simulink library "ECO_TestLibs"  (R2018a)
settings: Solver=ode45  StartTime=0.0  StopTime=10.0  RelTol=1e-3  EnableMultiTasking=on
undefined symbols (not defined in the file or in its folder): h, km
libraries: CoderSF_BSW_Libs x643, $bdroot x217, SF_CanService_Libs x60, simulink x12
(part 5 of 7)

== system ECO_TestLibs/TAF_TRI/FC_L50ms ==
  function : TriggerPort  TriggerType=function-call  VariantControl=(inherit)
  Display : Display
  GetPeriod_ms : $bdroot/GetPeriod_ms  frqP=TRI_frqFreeSys_val
  Write Measurement : CoderSF_BSW_Libs/Calibration & Measurement/Write Measurement  variable_name=TRI_tL50ms  variable_value=0  variable_type=single  numD=1  unitStr=ms  descStr=""
      settings: AttributesFormatString=value:%<variable_value> type:%<variable_type>  SourceProductName=EcoCoder Blocks
  dt : CoderSF_BSW_Libs/Application Base Blocks/dt
      settings: SourceProductName=EcoCoder Blocks
  wires:
  GetPeriod_ms/1 -> Write Measurement/1
  dt/1 -> Display/1

== system ECO_TestLibs/TAF_TRI/FC_L5ms ==
  function : TriggerPort  TriggerType=function-call  VariantControl=(inherit)
  Display : Display
  GetPeriod_ms : $bdroot/GetPeriod_ms  frqP=TRI_frqFreeSys_val
  Write Measurement : CoderSF_BSW_Libs/Calibration & Measurement/Write Measurement  variable_name=TRI_tL5ms  variable_value=0  variable_type=single  numD=1  unitStr=ms  descStr=""
      settings: AttributesFormatString=value:%<variable_value> type:%<variable_type>  SourceProductName=EcoCoder Blocks
  dt : CoderSF_BSW_Libs/Application Base Blocks/dt
      settings: SourceProductName=EcoCoder Blocks
  wires:
  GetPeriod_ms/1 -> Write Measurement/1
  dt/1 -> Display/1

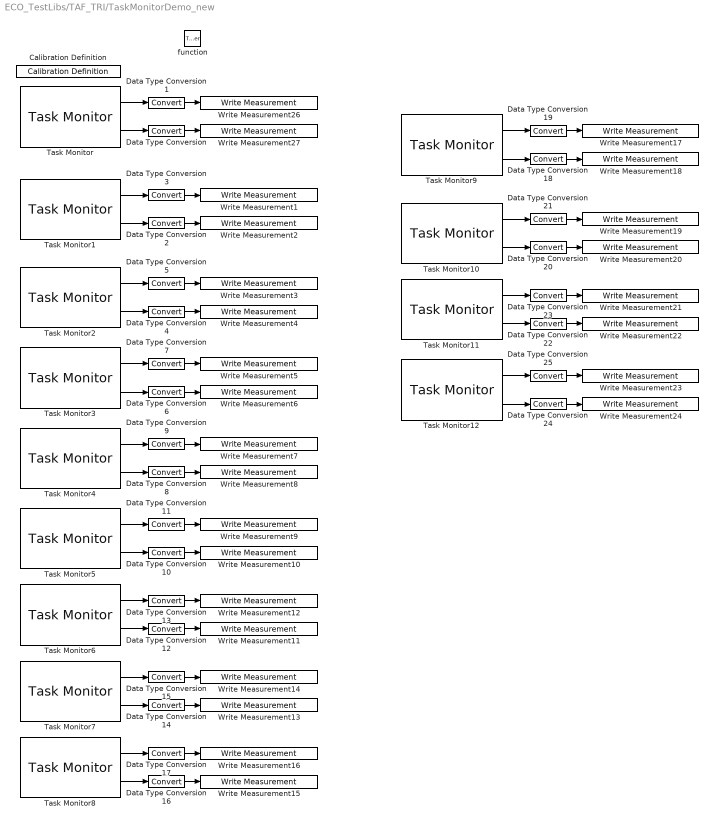
== system ECO_TestLibs/TAF_TRI/TaskMonitorDemo_new ==
  function : TriggerPort  TriggerType=function-call  VariantControl=(inherit)
  Calibration Definition : CoderSF_BSW_Libs/Calibration & Measurement/Calibration Definition  variable_name=MonitorNew_frqRTC_val  variable_value=5*1000  variable_type=single  variable_min=[]  variable_max=[]  unitStr=kHz  descStr=""
      settings: AttributesFormatString=value:%<variable_value> type:%<variable_type> max:%<variable_max> Min:%<variable_min>  SourceProductName=EcoCoder Blocks
  Data Type Conversion{,1..25} (26 alike) : DataTypeConversion  SaturateOnIntegerOverflow=on
  Task Monitor : CoderSF_BSW_Libs/Task Scheduler/Task Monitor  TasktimeIndex_Out=Task_L1ms  fac=MonitorNew_frqRTC_val
      settings: SourceProductName=EcoCoder Blocks
  Task Monitor1 : CoderSF_BSW_Libs/Task Scheduler/Task Monitor  TasktimeIndex_Out=Task_L5ms  fac=MonitorNew_frqRTC_val
      settings: SourceProductName=EcoCoder Blocks
  Task Monitor10 : CoderSF_BSW_Libs/Task Scheduler/Task Monitor  TasktimeIndex_Out=Task_H5ms  fac=MonitorNew_frqRTC_val
      settings: SourceProductName=EcoCoder Blocks
  Task Monitor11 : CoderSF_BSW_Libs/Task Scheduler/Task Monitor  TasktimeIndex_Out=Task_H10ms  fac=MonitorNew_frqRTC_val
      settings: SourceProductName=EcoCoder Blocks
  Task Monitor12 : CoderSF_BSW_Libs/Task Scheduler/Task Monitor  TasktimeIndex_Out=Task_H20ms  fac=MonitorNew_frqRTC_val
      settings: SourceProductName=EcoCoder Blocks
  Task Monitor2 : CoderSF_BSW_Libs/Task Scheduler/Task Monitor  TasktimeIndex_Out=Task_L10ms  fac=MonitorNew_frqRTC_val
      settings: SourceProductName=EcoCoder Blocks
  Task Monitor3 : CoderSF_BSW_Libs/Task Scheduler/Task Monitor  TasktimeIndex_Out=Task_L20ms  fac=MonitorNew_frqRTC_val
      settings: SourceProductName=EcoCoder Blocks
  Task Monitor4 : CoderSF_BSW_Libs/Task Scheduler/Task Monitor  TasktimeIndex_Out=Task_L50ms  fac=MonitorNew_frqRTC_val
      settings: SourceProductName=EcoCoder Blocks
  Task Monitor5 : CoderSF_BSW_Libs/Task Scheduler/Task Monitor  TasktimeIndex_Out=Task_L100ms  fac=MonitorNew_frqRTC_val
      settings: SourceProductName=EcoCoder Blocks
  Task Monitor6 : CoderSF_BSW_Libs/Task Scheduler/Task Monitor  TasktimeIndex_Out=Task_L200ms  fac=MonitorNew_frqRTC_val
      settings: SourceProductName=EcoCoder Blocks
  Task Monitor7 : CoderSF_BSW_Libs/Task Scheduler/Task Monitor  TasktimeIndex_Out=Task_L500ms  fac=MonitorNew_frqRTC_val
      settings: SourceProductName=EcoCoder Blocks
  Task Monitor8 : CoderSF_BSW_Libs/Task Scheduler/Task Monitor  TasktimeIndex_Out=Task_L1000ms  fac=MonitorNew_frqRTC_val
      settings: SourceProductName=EcoCoder Blocks
  Task Monitor9 : CoderSF_BSW_Libs/Task Scheduler/Task Monitor  TasktimeIndex_Out=Task_H1ms  fac=MonitorNew_frqRTC_val
      settings: SourceProductName=EcoCoder Blocks
  Write Measurement1 : CoderSF_BSW_Libs/Calibration & Measurement/Write Measurement  variable_name=MonitorNewL5ms_tI  variable_value=0  variable_type=fixdt(0,16,1/30,0)  numD=1  unitStr=ms  descStr=""
      settings: AttributesFormatString=type:%<variable_type> Dimensions:%<numD>  SourceProductName=EcoCoder Blocks
  Write Measurement10 : CoderSF_BSW_Libs/Calibration & Measurement/Write Measurement  variable_name=MonitorNewL100ms_pct  variable_value=0  variable_type=fixdt(0,8,100/255,0)  numD=1  unitStr=%  descStr=""
      settings: AttributesFormatString=type:%<variable_type> Dimensions:%<numD>  SourceProductName=EcoCoder Blocks
  Write Measurement11 : CoderSF_BSW_Libs/Calibration & Measurement/Write Measurement  variable_name=MonitorNewL200ms_pct  variable_value=0  variable_type=fixdt(0,8,100/255,0)  numD=1  unitStr=%  descStr=""
      settings: AttributesFormatString=type:%<variable_type> Dimensions:%<numD>  SourceProductName=EcoCoder Blocks
  Write Measurement12 : CoderSF_BSW_Libs/Calibration & Measurement/Write Measurement  variable_name=MonitorNewL200ms_tI  variable_value=0  variable_type=fixdt(0,16,1/30,0)  numD=1  unitStr=ms  descStr=""
      settings: AttributesFormatString=type:%<variable_type> Dimensions:%<numD>  SourceProductName=EcoCoder Blocks
  Write Measurement13 : CoderSF_BSW_Libs/Calibration & Measurement/Write Measurement  variable_name=MonitorNewL500ms_pct  variable_value=0  variable_type=fixdt(0,8,100/255,0)  numD=1  unitStr=%  descStr=""
      settings: AttributesFormatString=type:%<variable_type> Dimensions:%<numD>  SourceProductName=EcoCoder Blocks
  Write Measurement14 : CoderSF_BSW_Libs/Calibration & Measurement/Write Measurement  variable_name=MonitorNewL500ms_tI  variable_value=0  variable_type=fixdt(0,16,1/30,0)  numD=1  unitStr=ms  descStr=""
      settings: AttributesFormatString=type:%<variable_type> Dimensions:%<numD>  SourceProductName=EcoCoder Blocks
  Write Measurement15 : CoderSF_BSW_Libs/Calibration & Measurement/Write Measurement  variable_name=MonitorNewL1000ms_pct  variable_value=0  variable_type=fixdt(0,8,100/255,0)  numD=1  unitStr=%  descStr=""
      settings: AttributesFormatString=type:%<variable_type> Dimensions:%<numD>  SourceProductName=EcoCoder Blocks
  Write Measurement16 : CoderSF_BSW_Libs/Calibration & Measurement/Write Measurement  variable_name=MonitorNewL1000ms_tI  variable_value=0  variable_type=fixdt(0,16,1/30,0)  numD=1  unitStr=ms  descStr=""
      settings: AttributesFormatString=type:%<variable_type> Dimensions:%<numD>  SourceProductName=EcoCoder Blocks
  Write Measurement17 : CoderSF_BSW_Libs/Calibration & Measurement/Write Measurement  variable_name=MonitorNewH1ms_tI  variable_value=0  variable_type=fixdt(0,16,1/30,0)  numD=1  unitStr=ms  descStr=""
      settings: AttributesFormatString=type:%<variable_type> Dimensions:%<numD>  SourceProductName=EcoCoder Blocks
  Write Measurement18 : CoderSF_BSW_Libs/Calibration & Measurement/Write Measurement  variable_name=MonitorNewH1ms_pct  variable_value=0  variable_type=fixdt(0,8,100/255,0)  numD=1  unitStr=%  descStr=""
      settings: AttributesFormatString=type:%<variable_type> Dimensions:%<numD>  SourceProductName=EcoCoder Blocks
  Write Measurement19 : CoderSF_BSW_Libs/Calibration & Measurement/Write Measurement  variable_name=MonitorNewH5ms_tI  variable_value=0  variable_type=fixdt(0,16,1/30,0)  numD=1  unitStr=ms  descStr=""
      settings: AttributesFormatString=type:%<variable_type> Dimensions:%<numD>  SourceProductName=EcoCoder Blocks
  Write Measurement2 : CoderSF_BSW_Libs/Calibration & Measurement/Write Measurement  variable_name=MonitorNewL5ms_pct  variable_value=0  variable_type=fixdt(0,8,100/255,0)  numD=1  unitStr=%  descStr=""
      settings: AttributesFormatString=type:%<variable_type> Dimensions:%<numD>  SourceProductName=EcoCoder Blocks
  Write Measurement20 : CoderSF_BSW_Libs/Calibration & Measurement/Write Measurement  variable_name=MonitorNewH5ms_pct  variable_value=0  variable_type=fixdt(0,8,100/255,0)  numD=1  unitStr=%  descStr=""
      settings: AttributesFormatString=type:%<variable_type> Dimensions:%<numD>  SourceProductName=EcoCoder Blocks
  Write Measurement21 : CoderSF_BSW_Libs/Calibration & Measurement/Write Measurement  variable_name=MonitorNewH10ms_tI  variable_value=0  variable_type=fixdt(0,16,1/30,0)  numD=1  unitStr=ms  descStr=""
      settings: AttributesFormatString=type:%<variable_type> Dimensions:%<numD>  SourceProductName=EcoCoder Blocks
  Write Measurement22 : CoderSF_BSW_Libs/Calibration & Measurement/Write Measurement  variable_name=MonitorNewH10ms_pct  variable_value=0  variable_type=fixdt(0,8,100/255,0)  numD=1  unitStr=%  descStr=""
      settings: AttributesFormatString=type:%<variable_type> Dimensions:%<numD>  SourceProductName=EcoCoder Blocks
  Write Measurement23 : CoderSF_BSW_Libs/Calibration & Measurement/Write Measurement  variable_name=MonitorNewH20ms_tI  variable_value=0  variable_type=fixdt(0,16,1/30,0)  numD=1  unitStr=ms  descStr=""
      settings: AttributesFormatString=type:%<variable_type> Dimensions:%<numD>  SourceProductName=EcoCoder Blocks
  Write Measurement24 : CoderSF_BSW_Libs/Calibration & Measurement/Write Measurement  variable_name=MonitorNewH20ms_pct  variable_value=0  variable_type=fixdt(0,8,100/255,0)  numD=1  unitStr=%  descStr=""
      settings: AttributesFormatString=type:%<variable_type> Dimensions:%<numD>  SourceProductName=EcoCoder Blocks
  Write Measurement26 : CoderSF_BSW_Libs/Calibration & Measurement/Write Measurement  variable_name=MonitorNewL1ms_tI  variable_value=0  variable_type=fixdt(0,16,1/30,0)  numD=1  unitStr=ms  descStr=""
      settings: AttributesFormatString=type:%<variable_type> Dimensions:%<numD>  SourceProductName=EcoCoder Blocks
  Write Measurement27 : CoderSF_BSW_Libs/Calibration & Measurement/Write Measurement  variable_name=MonitorNewL1ms_pct  variable_value=0  variable_type=fixdt(0,8,100/255,0)  numD=1  unitStr=%  descStr=""
      settings: AttributesFormatString=type:%<variable_type> Dimensions:%<numD>  SourceProductName=EcoCoder Blocks
  Write Measurement3 : CoderSF_BSW_Libs/Calibration & Measurement/Write Measurement  variable_name=MonitorNewL10ms_tI  variable_value=0  variable_type=fixdt(0,16,1/30,0)  numD=1  unitStr=ms  descStr=""
      settings: AttributesFormatString=type:%<variable_type> Dimensions:%<numD>  SourceProductName=EcoCoder Blocks
  Write Measurement4 : CoderSF_BSW_Libs/Calibration & Measurement/Write Measurement  variable_name=MonitorNewL10ms_pct  variable_value=0  variable_type=fixdt(0,8,100/255,0)  numD=1  unitStr=%  descStr=""
      settings: AttributesFormatString=type:%<variable_type> Dimensions:%<numD>  SourceProductName=EcoCoder Blocks
  Write Measurement5 : CoderSF_BSW_Libs/Calibration & Measurement/Write Measurement  variable_name=MonitorNewL20ms_tI  variable_value=0  variable_type=fixdt(0,16,1/30,0)  numD=1  unitStr=ms  descStr=""
      settings: AttributesFormatString=type:%<variable_type> Dimensions:%<numD>  SourceProductName=EcoCoder Blocks
  Write Measurement6 : CoderSF_BSW_Libs/Calibration & Measurement/Write Measurement  variable_name=MonitorNewL20ms_pct  variable_value=0  variable_type=fixdt(0,8,100/255,0)  numD=1  unitStr=%  descStr=""
      settings: AttributesFormatString=type:%<variable_type> Dimensions:%<numD>  SourceProductName=EcoCoder Blocks
  Write Measurement7 : CoderSF_BSW_Libs/Calibration & Measurement/Write Measurement  variable_name=MonitorNewL50ms_tI  variable_value=0  variable_type=fixdt(0,16,1/30,0)  numD=1  unitStr=ms  descStr=""
      settings: AttributesFormatString=type:%<variable_type> Dimensions:%<numD>  SourceProductName=EcoCoder Blocks
  Write Measurement8 : CoderSF_BSW_Libs/Calibration & Measurement/Write Measurement  variable_name=MonitorNewL50ms_pct  variable_value=0  variable_type=fixdt(0,8,100/255,0)  numD=1  unitStr=%  descStr=""
      settings: AttributesFormatString=type:%<variable_type> Dimensions:%<numD>  SourceProductName=EcoCoder Blocks
  Write Measurement9 : CoderSF_BSW_Libs/Calibration & Measurement/Write Measurement  variable_name=MonitorNewL100ms_tI  variable_value=0  variable_type=fixdt(0,16,1/30,0)  numD=1  unitStr=ms  descStr=""
      settings: AttributesFormatString=type:%<variable_type> Dimensions:%<numD>  SourceProductName=EcoCoder Blocks
  wires:
  Task Monitor/1 -> Data Type Conversion1/1
  Task Monitor/2 -> Data Type Conversion/1
  Data Type Conversion/1 -> Write Measurement27/1
  Data Type Conversion1/1 -> Write Measurement26/1
  Task Monitor1/1 -> Data Type Conversion3/1
  Task Monitor1/2 -> Data Type Conversion2/1
  Data Type Conversion2/1 -> Write Measurement2/1
  Data Type Conversion3/1 -> Write Measurement1/1
  Task Monitor2/1 -> Data Type Conversion5/1
  Task Monitor2/2 -> Data Type Conversion4/1
  Data Type Conversion4/1 -> Write Measurement4/1
  Data Type Conversion5/1 -> Write Measurement3/1
  Task Monitor3/1 -> Data Type Conversion7/1
  Task Monitor3/2 -> Data Type Conversion6/1
  Data Type Conversion6/1 -> Write Measurement6/1
  Data Type Conversion7/1 -> Write Measurement5/1
  Task Monitor4/1 -> Data Type Conversion9/1
  Task Monitor4/2 -> Data Type Conversion8/1
  Data Type Conversion8/1 -> Write Measurement8/1
  Data Type Conversion9/1 -> Write Measurement7/1
  Task Monitor5/1 -> Data Type Conversion11/1
  Task Monitor5/2 -> Data Type Conversion10/1
  Data Type Conversion10/1 -> Write Measurement10/1
  Data Type Conversion11/1 -> Write Measurement9/1
  Task Monitor6/1 -> Data Type Conversion13/1
  Task Monitor6/2 -> Data Type Conversion12/1
  Data Type Conversion12/1 -> Write Measurement11/1
  Data Type Conversion13/1 -> Write Measurement12/1
  Task Monitor7/1 -> Data Type Conversion15/1
  Task Monitor7/2 -> Data Type Conversion14/1
  Data Type Conversion14/1 -> Write Measurement13/1
  Data Type Conversion15/1 -> Write Measurement14/1
  Task Monitor8/1 -> Data Type Conversion17/1
  Task Monitor8/2 -> Data Type Conversion16/1
  Data Type Conversion16/1 -> Write Measurement15/1
  Data Type Conversion17/1 -> Write Measurement16/1
  Task Monitor9/1 -> Data Type Conversion19/1
  Task Monitor9/2 -> Data Type Conversion18/1
  Data Type Conversion18/1 -> Write Measurement18/1
  Data Type Conversion19/1 -> Write Measurement17/1
  Task Monitor10/1 -> Data Type Conversion21/1
  Task Monitor10/2 -> Data Type Conversion20/1
  Data Type Conversion20/1 -> Write Measurement20/1
  Data Type Conversion21/1 -> Write Measurement19/1
  Task Monitor11/1 -> Data Type Conversion23/1
  Task Monitor11/2 -> Data Type Conversion22/1
  Data Type Conversion22/1 -> Write Measurement22/1
  Data Type Conversion23/1 -> Write Measurement21/1
  Task Monitor12/1 -> Data Type Conversion25/1
  Task Monitor12/2 -> Data Type Conversion24/1
  Data Type Conversion24/1 -> Write Measurement24/1
  Data Type Conversion25/1 -> Write Measurement23/1

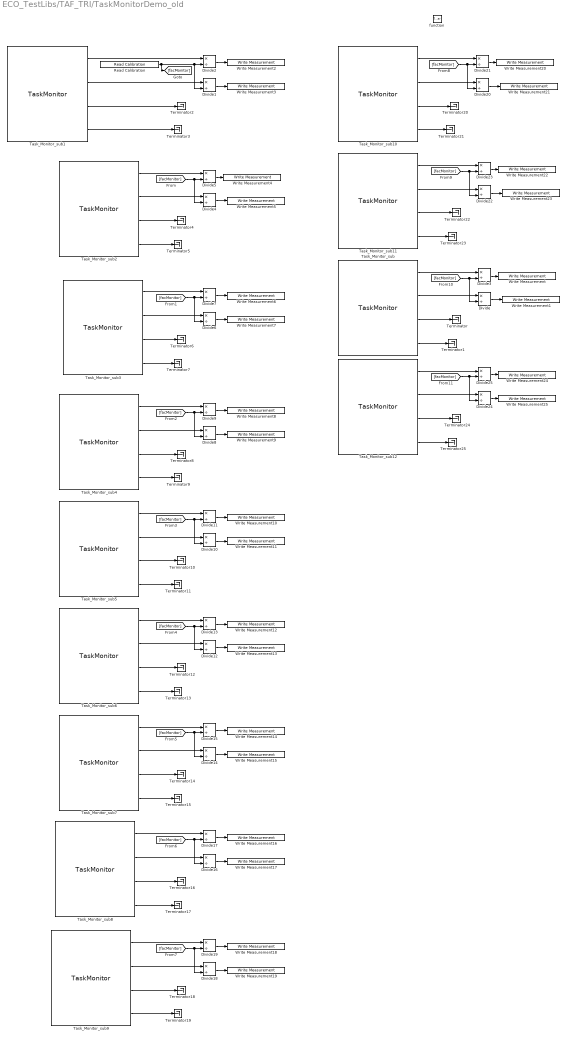
== system ECO_TestLibs/TAF_TRI/TaskMonitorDemo_old ==
  function : TriggerPort  TriggerType=function-call  VariantControl=(inherit)
  Divide{,1..25} (26 alike) : Product  Inputs=*/  OutDataTypeStr=single
  Read Calibration : CoderSF_BSW_Libs/Calibration & Measurement/Read Calibration  variable_name=Monitor_fac  variable_value=5*000  variable_type=single  variable_min=[]  variable_max=[]  unitStr=kHz  descStr=""
      settings: AttributesFormatString=value:%<variable_value> type:%<variable_type> max:%<variable_max> Min:%<variable_min>  SourceProductName=EcoCoder Blocks
  Task_Monitor_sub : S-Function  FunctionName=TaskMonitor  Parameters=tasktime*1000  SFunctionDeploymentMode=off  EnableBusSupport=off  mask{tasktimeIndex=Task_H10ms}
      mask prompts: tasktimeIndex "Task Timer Interface"
      mask init:
      | tasktime = scheduler_monitor_set(get_param(gcb,'tasktimeIndex'));
      | %disp(['task time:',num2str(tasktime)]);
      mask TypeOptions tasktimeIndex: Task_L1ms | Task_L5ms | Task_L10ms | Task_L20ms | Task_L50ms | Task_L100ms | Task_L200ms | Task_L500ms | Task_L1000ms | Task_H1ms | Task_H5ms | Task_H10ms | Task_H20ms
      mask Display:
      | EcoCoder_SkinColor;
      | disp(['Monitor:',get_param(gcb,'tasktimeIndex')]);
      | port_label('output',1,'tInterval');
      | port_label('output',2,'tConsume');
      | port_label('output',3,'tIntervalMax');
      | port_label('output',4,'tConsumeMax');
  Task_Monitor_sub1 : S-Function  FunctionName=TaskMonitor  Parameters=tasktime*1000  SFunctionDeploymentMode=off  EnableBusSupport=off  mask{tasktimeIndex=Task_L1ms}
      mask prompts: tasktimeIndex "Task Timer Interface"
      mask init:
      | tasktime = scheduler_monitor_set(get_param(gcb,'tasktimeIndex'));
      | %disp(['task time:',num2str(tasktime)]);
      mask TypeOptions tasktimeIndex: Task_L1ms | Task_L5ms | Task_L10ms | Task_L20ms | Task_L50ms | Task_L100ms | Task_L200ms | Task_L500ms | Task_L1000ms | Task_H1ms | Task_H5ms | Task_H10ms | Task_H20ms
      mask Display:
      | EcoCoder_SkinColor;
      | disp(['Monitor:',get_param(gcb,'tasktimeIndex')]);
      | port_label('output',1,'tInterval');
      | port_label('output',2,'tConsume');
      | port_label('output',3,'tIntervalMax');
      | port_label('output',4,'tConsumeMax');
  Task_Monitor_sub10 : S-Function  FunctionName=TaskMonitor  Parameters=tasktime*1000  SFunctionDeploymentMode=off  EnableBusSupport=off  mask{tasktimeIndex=Task_H1ms}
      mask prompts: tasktimeIndex "Task Timer Interface"
      mask init:
      | tasktime = scheduler_monitor_set(get_param(gcb,'tasktimeIndex'));
      | %disp(['task time:',num2str(tasktime)]);
      mask TypeOptions tasktimeIndex: Task_L1ms | Task_L5ms | Task_L10ms | Task_L20ms | Task_L50ms | Task_L100ms | Task_L200ms | Task_L500ms | Task_L1000ms | Task_H1ms | Task_H5ms | Task_H10ms | Task_H20ms
      mask Display:
      | EcoCoder_SkinColor;
      | disp(['Monitor:',get_param(gcb,'tasktimeIndex')]);
      | port_label('output',1,'tInterval');
      | port_label('output',2,'tConsume');
      | port_label('output',3,'tIntervalMax');
      | port_label('output',4,'tConsumeMax');
  Task_Monitor_sub11 : S-Function  FunctionName=TaskMonitor  Parameters=tasktime*1000  SFunctionDeploymentMode=off  EnableBusSupport=off  mask{tasktimeIndex=Task_H5ms}
      mask prompts: tasktimeIndex "Task Timer Interface"
      mask init:
      | tasktime = scheduler_monitor_set(get_param(gcb,'tasktimeIndex'));
      | %disp(['task time:',num2str(tasktime)]);
      mask TypeOptions tasktimeIndex: Task_L1ms | Task_L5ms | Task_L10ms | Task_L20ms | Task_L50ms | Task_L100ms | Task_L200ms | Task_L500ms | Task_L1000ms | Task_H1ms | Task_H5ms | Task_H10ms | Task_H20ms
      mask Display:
      | EcoCoder_SkinColor;
      | disp(['Monitor:',get_param(gcb,'tasktimeIndex')]);
      | port_label('output',1,'tInterval');
      | port_label('output',2,'tConsume');
      | port_label('output',3,'tIntervalMax');
      | port_label('output',4,'tConsumeMax');
  Task_Monitor_sub12 : S-Function  FunctionName=TaskMonitor  Parameters=tasktime*1000  SFunctionDeploymentMode=off  EnableBusSupport=off  mask{tasktimeIndex=Task_H20ms}
      mask prompts: tasktimeIndex "Task Timer Interface"
      mask init:
      | tasktime = scheduler_monitor_set(get_param(gcb,'tasktimeIndex'));
      | %disp(['task time:',num2str(tasktime)]);
      mask TypeOptions tasktimeIndex: Task_L1ms | Task_L5ms | Task_L10ms | Task_L20ms | Task_L50ms | Task_L100ms | Task_L200ms | Task_L500ms | Task_L1000ms | Task_H1ms | Task_H5ms | Task_H10ms | Task_H20ms
      mask Display:
      | EcoCoder_SkinColor;
      | disp(['Monitor:',get_param(gcb,'tasktimeIndex')]);
      | port_label('output',1,'tInterval');
      | port_label('output',2,'tConsume');
      | port_label('output',3,'tIntervalMax');
      | port_label('output',4,'tConsumeMax');
  Task_Monitor_sub2 : S-Function  FunctionName=TaskMonitor  Parameters=tasktime*1000  SFunctionDeploymentMode=off  EnableBusSupport=off  mask{tasktimeIndex=Task_L5ms}
      mask prompts: tasktimeIndex "Task Timer Interface"
      mask init:
      | tasktime = scheduler_monitor_set(get_param(gcb,'tasktimeIndex'));
      | %disp(['task time:',num2str(tasktime)]);
      mask TypeOptions tasktimeIndex: Task_L1ms | Task_L5ms | Task_L10ms | Task_L20ms | Task_L50ms | Task_L100ms | Task_L200ms | Task_L500ms | Task_L1000ms | Task_H1ms | Task_H5ms | Task_H10ms | Task_H20ms
      mask Display:
      | EcoCoder_SkinColor;
      | disp(['Monitor:',get_param(gcb,'tasktimeIndex')]);
      | port_label('output',1,'tInterval');
      | port_label('output',2,'tConsume');
      | port_label('output',3,'tIntervalMax');
      | port_label('output',4,'tConsumeMax');
  Task_Monitor_sub3 : S-Function  FunctionName=TaskMonitor  Parameters=tasktime*1000  SFunctionDeploymentMode=off  EnableBusSupport=off  mask{tasktimeIndex=Task_L10ms}
      mask prompts: tasktimeIndex "Task Timer Interface"
      mask init:
      | tasktime = scheduler_monitor_set(get_param(gcb,'tasktimeIndex'));
      | %disp(['task time:',num2str(tasktime)]);
      mask TypeOptions tasktimeIndex: Task_L1ms | Task_L5ms | Task_L10ms | Task_L20ms | Task_L50ms | Task_L100ms | Task_L200ms | Task_L500ms | Task_L1000ms | Task_H1ms | Task_H5ms | Task_H10ms | Task_H20ms
      mask Display:
      | EcoCoder_SkinColor;
      | disp(['Monitor:',get_param(gcb,'tasktimeIndex')]);
      | port_label('output',1,'tInterval');
      | port_label('output',2,'tConsume');
      | port_label('output',3,'tIntervalMax');
      | port_label('output',4,'tConsumeMax');
  Task_Monitor_sub4 : S-Function  FunctionName=TaskMonitor  Parameters=tasktime*1000  SFunctionDeploymentMode=off  EnableBusSupport=off  mask{tasktimeIndex=Task_L20ms}
      mask prompts: tasktimeIndex "Task Timer Interface"
      mask init:
      | tasktime = scheduler_monitor_set(get_param(gcb,'tasktimeIndex'));
      | %disp(['task time:',num2str(tasktime)]);
      mask TypeOptions tasktimeIndex: Task_L1ms | Task_L5ms | Task_L10ms | Task_L20ms | Task_L50ms | Task_L100ms | Task_L200ms | Task_L500ms | Task_L1000ms | Task_H1ms | Task_H5ms | Task_H10ms | Task_H20ms
      mask Display:
      | EcoCoder_SkinColor;
      | disp(['Monitor:',get_param(gcb,'tasktimeIndex')]);
      | port_label('output',1,'tInterval');
      | port_label('output',2,'tConsume');
      | port_label('output',3,'tIntervalMax');
      | port_label('output',4,'tConsumeMax');
  Task_Monitor_sub5 : S-Function  FunctionName=TaskMonitor  Parameters=tasktime*1000  SFunctionDeploymentMode=off  EnableBusSupport=off  mask{tasktimeIndex=Task_L50ms}
      mask prompts: tasktimeIndex "Task Timer Interface"
      mask init:
      | tasktime = scheduler_monitor_set(get_param(gcb,'tasktimeIndex'));
      | %disp(['task time:',num2str(tasktime)]);
      mask TypeOptions tasktimeIndex: Task_L1ms | Task_L5ms | Task_L10ms | Task_L20ms | Task_L50ms | Task_L100ms | Task_L200ms | Task_L500ms | Task_L1000ms | Task_H1ms | Task_H5ms | Task_H10ms | Task_H20ms
      mask Display:
      | EcoCoder_SkinColor;
      | disp(['Monitor:',get_param(gcb,'tasktimeIndex')]);
      | port_label('output',1,'tInterval');
      | port_label('output',2,'tConsume');
      | port_label('output',3,'tIntervalMax');
      | port_label('output',4,'tConsumeMax');
  Task_Monitor_sub6 : S-Function  FunctionName=TaskMonitor  Parameters=tasktime*1000  SFunctionDeploymentMode=off  EnableBusSupport=off  mask{tasktimeIndex=Task_L100ms}
      mask prompts: tasktimeIndex "Task Timer Interface"
      mask init:
      | tasktime = scheduler_monitor_set(get_param(gcb,'tasktimeIndex'));
      | %disp(['task time:',num2str(tasktime)]);
      mask TypeOptions tasktimeIndex: Task_L1ms | Task_L5ms | Task_L10ms | Task_L20ms | Task_L50ms | Task_L100ms | Task_L200ms | Task_L500ms | Task_L1000ms | Task_H1ms | Task_H5ms | Task_H10ms | Task_H20ms
      mask Display:
      | EcoCoder_SkinColor;
      | disp(['Monitor:',get_param(gcb,'tasktimeIndex')]);
      | port_label('output',1,'tInterval');
      | port_label('output',2,'tConsume');
      | port_label('output',3,'tIntervalMax');
      | port_label('output',4,'tConsumeMax');
  Task_Monitor_sub7 : S-Function  FunctionName=TaskMonitor  Parameters=tasktime*1000  SFunctionDeploymentMode=off  EnableBusSupport=off  mask{tasktimeIndex=Task_L200ms}
      mask prompts: tasktimeIndex "Task Timer Interface"
      mask init:
      | tasktime = scheduler_monitor_set(get_param(gcb,'tasktimeIndex'));
      | %disp(['task time:',num2str(tasktime)]);
      mask TypeOptions tasktimeIndex: Task_L1ms | Task_L5ms | Task_L10ms | Task_L20ms | Task_L50ms | Task_L100ms | Task_L200ms | Task_L500ms | Task_L1000ms | Task_H1ms | Task_H5ms | Task_H10ms | Task_H20ms
      mask Display:
      | EcoCoder_SkinColor;
      | disp(['Monitor:',get_param(gcb,'tasktimeIndex')]);
      | port_label('output',1,'tInterval');
      | port_label('output',2,'tConsume');
      | port_label('output',3,'tIntervalMax');
      | port_label('output',4,'tConsumeMax');
  Task_Monitor_sub8 : S-Function  FunctionName=TaskMonitor  Parameters=tasktime*1000  SFunctionDeploymentMode=off  EnableBusSupport=off  mask{tasktimeIndex=Task_L500ms}
      mask prompts: tasktimeIndex "Task Timer Interface"
      mask init:
      | tasktime = scheduler_monitor_set(get_param(gcb,'tasktimeIndex'));
      | %disp(['task time:',num2str(tasktime)]);
      mask TypeOptions tasktimeIndex: Task_L1ms | Task_L5ms | Task_L10ms | Task_L20ms | Task_L50ms | Task_L100ms | Task_L200ms | Task_L500ms | Task_L1000ms | Task_H1ms | Task_H5ms | Task_H10ms | Task_H20ms
      mask Display:
      | EcoCoder_SkinColor;
      | disp(['Monitor:',get_param(gcb,'tasktimeIndex')]);
      | port_label('output',1,'tInterval');
      | port_label('output',2,'tConsume');
      | port_label('output',3,'tIntervalMax');
      | port_label('output',4,'tConsumeMax');
  Task_Monitor_sub9 : S-Function  FunctionName=TaskMonitor  Parameters=tasktime*1000  SFunctionDeploymentMode=off  EnableBusSupport=off  mask{tasktimeIndex=Task_L1000ms}
      mask prompts: tasktimeIndex "Task Timer Interface"
      mask init:
      | tasktime = scheduler_monitor_set(get_param(gcb,'tasktimeIndex'));
      | %disp(['task time:',num2str(tasktime)]);
      mask TypeOptions tasktimeIndex: Task_L1ms | Task_L5ms | Task_L10ms | Task_L20ms | Task_L50ms | Task_L100ms | Task_L200ms | Task_L500ms | Task_L1000ms | Task_H1ms | Task_H5ms | Task_H10ms | Task_H20ms
      mask Display:
      | EcoCoder_SkinColor;
      | disp(['Monitor:',get_param(gcb,'tasktimeIndex')]);
      | port_label('output',1,'tInterval');
      | port_label('output',2,'tConsume');
      | port_label('output',3,'tIntervalMax');
      | port_label('output',4,'tConsumeMax');
  Terminator{,1..25} (26 alike) : Terminator
  Write Measurement : CoderSF_BSW_Libs/Calibration & Measurement/Write Measurement  variable_name=MonitorH10ms_tI  variable_value=0  variable_type=single  numD=1  unitStr=ms  descStr=""
      settings: AttributesFormatString=type:%<variable_type> Dimensions:%<numD>  SourceProductName=EcoCoder Blocks
  Write Measurement1 : CoderSF_BSW_Libs/Calibration & Measurement/Write Measurement  variable_name=MonitorH10ms_tC  variable_value=0  variable_type=single  numD=1  unitStr=ms  descStr=""
      settings: AttributesFormatString=type:%<variable_type> Dimensions:%<numD>  SourceProductName=EcoCoder Blocks
  Write Measurement10 : CoderSF_BSW_Libs/Calibration & Measurement/Write Measurement  variable_name=MonitorL50ms_tI  variable_value=0  variable_type=single  numD=1  unitStr=ms  descStr=""
      settings: AttributesFormatString=type:%<variable_type> Dimensions:%<numD>  SourceProductName=EcoCoder Blocks
  Write Measurement11 : CoderSF_BSW_Libs/Calibration & Measurement/Write Measurement  variable_name=MonitorL50ms_tC  variable_value=0  variable_type=single  numD=1  unitStr=ms  descStr=""
      settings: AttributesFormatString=type:%<variable_type> Dimensions:%<numD>  SourceProductName=EcoCoder Blocks
  Write Measurement12 : CoderSF_BSW_Libs/Calibration & Measurement/Write Measurement  variable_name=MonitorL100ms_tI  variable_value=0  variable_type=single  numD=1  unitStr=ms  descStr=""
      settings: AttributesFormatString=type:%<variable_type> Dimensions:%<numD>  SourceProductName=EcoCoder Blocks
  Write Measurement13 : CoderSF_BSW_Libs/Calibration & Measurement/Write Measurement  variable_name=MonitorL100ms_tC  variable_value=0  variable_type=single  numD=1  unitStr=ms  descStr=""
      settings: AttributesFormatString=type:%<variable_type> Dimensions:%<numD>  SourceProductName=EcoCoder Blocks
  Write Measurement14 : CoderSF_BSW_Libs/Calibration & Measurement/Write Measurement  variable_name=MonitorL200ms_tI  variable_value=0  variable_type=single  numD=1  unitStr=ms  descStr=""
      settings: AttributesFormatString=type:%<variable_type> Dimensions:%<numD>  SourceProductName=EcoCoder Blocks
  Write Measurement15 : CoderSF_BSW_Libs/Calibration & Measurement/Write Measurement  variable_name=MonitorL200ms_tC  variable_value=0  variable_type=single  numD=1  unitStr=ms  descStr=""
      settings: AttributesFormatString=type:%<variable_type> Dimensions:%<numD>  SourceProductName=EcoCoder Blocks
  Write Measurement16 : CoderSF_BSW_Libs/Calibration & Measurement/Write Measurement  variable_name=MonitorL500ms_tI  variable_value=0  variable_type=single  numD=1  unitStr=ms  descStr=""
      settings: AttributesFormatString=type:%<variable_type> Dimensions:%<numD>  SourceProductName=EcoCoder Blocks
  Write Measurement17 : CoderSF_BSW_Libs/Calibration & Measurement/Write Measurement  variable_name=MonitorL500ms_tC  variable_value=0  variable_type=single  numD=1  unitStr=ms  descStr=""
      settings: AttributesFormatString=type:%<variable_type> Dimensions:%<numD>  SourceProductName=EcoCoder Blocks
  Write Measurement18 : CoderSF_BSW_Libs/Calibration & Measurement/Write Measurement  variable_name=MonitorL1000ms_tI  variable_value=0  variable_type=single  numD=1  unitStr=ms  descStr=""
      settings: AttributesFormatString=type:%<variable_type> Dimensions:%<numD>  SourceProductName=EcoCoder Blocks
  Write Measurement19 : CoderSF_BSW_Libs/Calibration & Measurement/Write Measurement  variable_name=MonitorL1000ms_tC  variable_value=0  variable_type=single  numD=1  unitStr=ms  descStr=""
      settings: AttributesFormatString=type:%<variable_type> Dimensions:%<numD>  SourceProductName=EcoCoder Blocks
  Write Measurement2 : CoderSF_BSW_Libs/Calibration & Measurement/Write Measurement  variable_name=MonitorL1ms_tI  variable_value=0  variable_type=single  numD=1  unitStr=ms  descStr=""
      settings: AttributesFormatString=type:%<variable_type> Dimensions:%<numD>  SourceProductName=EcoCoder Blocks
  Write Measurement20 : CoderSF_BSW_Libs/Calibration & Measurement/Write Measurement  variable_name=MonitorH1ms_tI  variable_value=0  variable_type=single  numD=1  unitStr=ms  descStr=""
      settings: AttributesFormatString=type:%<variable_type> Dimensions:%<numD>  SourceProductName=EcoCoder Blocks
  Write Measurement21 : CoderSF_BSW_Libs/Calibration & Measurement/Write Measurement  variable_name=MonitorH1ms_tC  variable_value=0  variable_type=single  numD=1  unitStr=ms  descStr=""
      settings: AttributesFormatString=type:%<variable_type> Dimensions:%<numD>  SourceProductName=EcoCoder Blocks
  Write Measurement22 : CoderSF_BSW_Libs/Calibration & Measurement/Write Measurement  variable_name=MonitorH5ms_tI  variable_value=0  variable_type=single  numD=1  unitStr=ms  descStr=""
      settings: AttributesFormatString=type:%<variable_type> Dimensions:%<numD>  SourceProductName=EcoCoder Blocks
  Write Measurement23 : CoderSF_BSW_Libs/Calibration & Measurement/Write Measurement  variable_name=MonitorH5ms_tC  variable_value=0  variable_type=single  numD=1  unitStr=ms  descStr=""
      settings: AttributesFormatString=type:%<variable_type> Dimensions:%<numD>  SourceProductName=EcoCoder Blocks
  Write Measurement24 : CoderSF_BSW_Libs/Calibration & Measurement/Write Measurement  variable_name=MonitorH20ms_tI  variable_value=0  variable_type=single  numD=1  unitStr=ms  descStr=""
      settings: AttributesFormatString=type:%<variable_type> Dimensions:%<numD>  SourceProductName=EcoCoder Blocks
  Write Measurement25 : CoderSF_BSW_Libs/Calibration & Measurement/Write Measurement  variable_name=MonitorH20ms_tC  variable_value=0  variable_type=single  numD=1  unitStr=ms  descStr=""
      settings: AttributesFormatString=type:%<variable_type> Dimensions:%<numD>  SourceProductName=EcoCoder Blocks
  Write Measurement3 : CoderSF_BSW_Libs/Calibration & Measurement/Write Measurement  variable_name=MonitorL1ms_tC  variable_value=0  variable_type=single  numD=1  unitStr=ms  descStr=""
      settings: AttributesFormatString=type:%<variable_type> Dimensions:%<numD>  SourceProductName=EcoCoder Blocks
  Write Measurement4 : CoderSF_BSW_Libs/Calibration & Measurement/Write Measurement  variable_name=MonitorL5ms_tI  variable_value=0  variable_type=single  numD=1  unitStr=ms  descStr=""
      settings: AttributesFormatString=type:%<variable_type> Dimensions:%<numD>  SourceProductName=EcoCoder Blocks
  Write Measurement5 : CoderSF_BSW_Libs/Calibration & Measurement/Write Measurement  variable_name=MonitorL5ms_tC  variable_value=0  variable_type=single  numD=1  unitStr=ms  descStr=""
      settings: AttributesFormatString=type:%<variable_type> Dimensions:%<numD>  SourceProductName=EcoCoder Blocks
  Write Measurement6 : CoderSF_BSW_Libs/Calibration & Measurement/Write Measurement  variable_name=MonitorL10ms_tI  variable_value=0  variable_type=single  numD=1  unitStr=ms  descStr=""
      settings: AttributesFormatString=type:%<variable_type> Dimensions:%<numD>  SourceProductName=EcoCoder Blocks
  Write Measurement7 : CoderSF_BSW_Libs/Calibration & Measurement/Write Measurement  variable_name=MonitorL10ms_tC  variable_value=0  variable_type=single  numD=1  unitStr=ms  descStr=""
      settings: AttributesFormatString=type:%<variable_type> Dimensions:%<numD>  SourceProductName=EcoCoder Blocks
  Write Measurement8 : CoderSF_BSW_Libs/Calibration & Measurement/Write Measurement  variable_name=MonitorL20ms_tI  variable_value=0  variable_type=single  numD=1  unitStr=ms  descStr=""
      settings: AttributesFormatString=type:%<variable_type> Dimensions:%<numD>  SourceProductName=EcoCoder Blocks
  Write Measurement9 : CoderSF_BSW_Libs/Calibration & Measurement/Write Measurement  variable_name=MonitorL20ms_tC  variable_value=0  variable_type=single  numD=1  unitStr=ms  descStr=""
      settings: AttributesFormatString=type:%<variable_type> Dimensions:%<numD>  SourceProductName=EcoCoder Blocks
  wires:
  Task_Monitor_sub/4 -> Terminator1/1
  Task_Monitor_sub/3 -> Terminator/1
  [facMonitor] -> Divide/2, Divide3/2
  Divide3/1 -> Write Measurement/1
  Task_Monitor_sub/1 -> Divide3/1
  Task_Monitor_sub/2 -> Divide/1
  Divide/1 -> Write Measurement1/1
  Task_Monitor_sub1/4 -> Terminator3/1
  Task_Monitor_sub1/3 -> Terminator2/1
  Read Calibration/1 -> Divide2/2, Divide1/2, [facMonitor]
  Divide2/1 -> Write Measurement2/1
  Task_Monitor_sub1/1 -> Divide2/1
  Task_Monitor_sub1/2 -> Divide1/1
  Divide1/1 -> Write Measurement3/1
  Task_Monitor_sub2/4 -> Terminator5/1
  Task_Monitor_sub2/3 -> Terminator4/1
  [facMonitor] -> Divide4/2, Divide5/2
  Divide5/1 -> Write Measurement4/1
  Task_Monitor_sub2/1 -> Divide5/1
  Task_Monitor_sub2/2 -> Divide4/1
  Divide4/1 -> Write Measurement5/1
  Task_Monitor_sub3/4 -> Terminator7/1
  Task_Monitor_sub3/3 -> Terminator6/1
  [facMonitor] -> Divide7/2, Divide6/2
  Divide7/1 -> Write Measurement6/1
  Task_Monitor_sub3/1 -> Divide7/1
  Task_Monitor_sub3/2 -> Divide6/1
  Divide6/1 -> Write Measurement7/1
  Task_Monitor_sub4/4 -> Terminator9/1
  Task_Monitor_sub4/3 -> Terminator8/1
  [facMonitor] -> Divide8/2, Divide9/2
  Divide9/1 -> Write Measurement8/1
  Task_Monitor_sub4/1 -> Divide9/1
  Task_Monitor_sub4/2 -> Divide8/1
  Divide8/1 -> Write Measurement9/1
  Task_Monitor_sub5/4 -> Terminator11/1
  Task_Monitor_sub5/3 -> Terminator10/1
  [facMonitor] -> Divide11/2, Divide10/2
  Divide11/1 -> Write Measurement10/1
  Task_Monitor_sub5/1 -> Divide11/1
  Task_Monitor_sub5/2 -> Divide10/1
  Divide10/1 -> Write Measurement11/1
  Task_Monitor_sub6/4 -> Terminator13/1
  Task_Monitor_sub6/3 -> Terminator12/1
  [facMonitor] -> Divide12/2, Divide13/2
  Divide13/1 -> Write Measurement12/1
  Task_Monitor_sub6/1 -> Divide13/1
  Task_Monitor_sub6/2 -> Divide12/1
  Divide12/1 -> Write Measurement13/1
  Task_Monitor_sub7/4 -> Terminator15/1
  Task_Monitor_sub7/3 -> Terminator14/1
  [facMonitor] -> Divide15/2, Divide14/2
  Divide15/1 -> Write Measurement14/1
  Task_Monitor_sub7/1 -> Divide15/1
  Task_Monitor_sub7/2 -> Divide14/1
  Divide14/1 -> Write Measurement15/1
  Task_Monitor_sub8/4 -> Terminator17/1
  Task_Monitor_sub8/3 -> Terminator16/1
  [facMonitor] -> Divide16/2, Divide17/2
  Divide17/1 -> Write Measurement16/1
  Task_Monitor_sub8/1 -> Divide17/1
  Task_Monitor_sub8/2 -> Divide16/1
  Divide16/1 -> Write Measurement17/1
  Task_Monitor_sub9/4 -> Terminator19/1
  Task_Monitor_sub9/3 -> Terminator18/1
  [facMonitor] -> Divide19/2, Divide18/2
  Divide19/1 -> Write Measurement18/1
  Task_Monitor_sub9/1 -> Divide19/1
  Task_Monitor_sub9/2 -> Divide18/1
  Divide18/1 -> Write Measurement19/1
  Task_Monitor_sub10/4 -> Terminator21/1
  Task_Monitor_sub10/3 -> Terminator20/1
  [facMonitor] -> Divide21/2, Divide20/2
  Divide21/1 -> Write Measurement20/1
  Task_Monitor_sub10/1 -> Divide21/1
  Task_Monitor_sub10/2 -> Divide20/1
  Divide20/1 -> Write Measurement21/1
  Task_Monitor_sub11/4 -> Terminator23/1
  Task_Monitor_sub11/3 -> Terminator22/1
  [facMonitor] -> Divide23/2, Divide22/2
  Divide23/1 -> Write Measurement22/1
  Task_Monitor_sub11/1 -> Divide23/1
  Task_Monitor_sub11/2 -> Divide22/1
  Divide22/1 -> Write Measurement23/1
  Task_Monitor_sub12/4 -> Terminator25/1
  Task_Monitor_sub12/3 -> Terminator24/1
  [facMonitor] -> Divide25/2, Divide24/2
  Divide25/1 -> Write Measurement24/1
  Task_Monitor_sub12/1 -> Divide25/1
  Task_Monitor_sub12/2 -> Divide24/1
  Divide24/1 -> Write Measurement25/1

== system ECO_TestLibs/TAF_TRI/Test_DeadWhile_H1m ==
  function : TriggerPort  TriggerType=function-call  VariantControl=(inherit)
  Function-Call Subsystem : Subsystem  TreatAsAtomicUnit=on
  While Function Only Code : S-Function  FunctionName=ecocoder_sf_while  SFunctionDeploymentMode=off  EnableBusSupport=off  mask(While Function Only Code){}
      mask help: While Function Only Code
      mask Display: disp('While Function Only Code');
  Write Measurement : CoderSF_BSW_Libs/Calibration & Measurement/Write Measurement  variable_name=TRI_flgDeadWhileH1mV  variable_value=0  variable_type=boolean  numD=1  unitStr=""  descStr=""
      settings: AttributesFormatString=value:%<variable_value> type:%<variable_type>  SourceProductName=EcoCoder Blocks
  ecocoder_calibration : CoderSF_BSW_Libs/Calibration & Measurement/Read Calibration  variable_name=TRI_flgDeadWhileH1m_val  variable_value=0  variable_type=boolean  variable_min=[]  variable_max=[]  unitStr=""  descStr=""
      settings: AttributesFormatString=value:%<variable_value> type:%<variable_type> max:%<variable_max> Min:%<variable_min>  SourceProductName=EcoCoder Blocks
  ecocoder_measurement : CoderSF_BSW_Libs/Calibration & Measurement/Write and Read Measurement  variable_name=TRI_flgDeadWhileH1m  variable_value=0  variable_type=boolean  numD=1  unitStr=""  descStr=""
      settings: AttributesFormatString=value:%<variable_value> type:%<variable_type>  SourceProductName=EcoCoder Blocks
  wires:
  ecocoder_calibration/1 -> ecocoder_measurement/1
  ecocoder_measurement/1 -> Function-Call Subsystem/1(In1), While Function Only Code/1
  While Function Only Code/1 -> Function-Call Subsystem/Trigger
  Function-Call Subsystem/1(Out1) -> Write Measurement/1

== system ECO_TestLibs/TAF_TRI/Test_DeadWhile_L1m ==
  function : TriggerPort  TriggerType=function-call  VariantControl=(inherit)
  Function-Call Subsystem : Subsystem  TreatAsAtomicUnit=on
  While Function Only Code : S-Function  FunctionName=ecocoder_sf_while  SFunctionDeploymentMode=off  EnableBusSupport=off  mask(While Function Only Code){}
      mask help: While Function Only Code
      mask Display: disp('While Function Only Code');
  Write Measurement : CoderSF_BSW_Libs/Calibration & Measurement/Write Measurement  variable_name=TRI_flgDeadWhileL1mV  variable_value=0  variable_type=boolean  numD=1  unitStr=""  descStr=""
      settings: AttributesFormatString=value:%<variable_value> type:%<variable_type>  SourceProductName=EcoCoder Blocks
  ecocoder_calibration : CoderSF_BSW_Libs/Calibration & Measurement/Read Calibration  variable_name=TRI_flgDeadWhileL1m_val  variable_value=0  variable_type=boolean  variable_min=[]  variable_max=[]  unitStr=""  descStr=""
      settings: AttributesFormatString=value:%<variable_value> type:%<variable_type> max:%<variable_max> Min:%<variable_min>  SourceProductName=EcoCoder Blocks
  ecocoder_measurement : CoderSF_BSW_Libs/Calibration & Measurement/Write and Read Measurement  variable_name=TRI_flgDeadWhileL1m  variable_value=0  variable_type=boolean  numD=1  unitStr=""  descStr=""
      settings: AttributesFormatString=value:%<variable_value> type:%<variable_type>  SourceProductName=EcoCoder Blocks
  wires:
  ecocoder_measurement/1 -> Function-Call Subsystem/1(In1), While Function Only Code/1
  ecocoder_calibration/1 -> ecocoder_measurement/1
  While Function Only Code/1 -> Function-Call Subsystem/Trigger
  Function-Call Subsystem/1(Out1) -> Write Measurement/1

== system ECO_TestLibs/LINAMaster/RTX/Delay2 ==
  z-1 : Inport
  Rising : Inport  Port=2
  Constant : Constant  Value=0  OutDataTypeStr=Inherit: Inherit via back propagation
  Rising Edge : Subsystem  TreatAsAtomicUnit=on  mask(Rising Edge){InitialCondition=on}
      mask prompts: InitialCondition "Initial Condition is true"
      mask help: Rising Edge
      settings: RTWSystemCode=Inline
      mask Display:
      | EcoCoder_SkinColor;
      | plot([0.1 0.5 0.5 0.9],[0.1 0.1 0.9 0.9])
      | plot([0.4 0.5 0.6],[0.45 0.6 0.45])
  Switch : Switch  Criteria=u2 ~= 0
  Unit Delay : UnitDelay  SampleTime=-1
  " " : Outport
  wires:
  z-1/1 -> Unit Delay/1
  Constant/1 -> Switch/1
  Rising Edge/1(out) -> Switch/2
  Rising/1 -> Rising Edge/1(in)
  Switch/1 -> " "/1
  Unit Delay/1 -> Switch/3

== system ECO_TestLibs/LINAMaster/RTX/Mst Rx Mod ==
  Enable : EnablePort
  LIN Receive Data1 : CoderSF_BSW_Libs/LIN/LIN Receive Data  channel=LIN_A  Frame_Id=hex2dec('4')  Frame_Len=8  Frame_Dir=MasterReceive  Frame_CCS=Classic  Task_TimeIdx=Task_Inherit
      settings: SourceProductName=EcoCoder Blocks
  Subsystem : Subsystem
  Write and Read Measurement : CoderSF_BSW_Libs/Calibration & Measurement/Write and Read Measurement  variable_name=LIN_Id4_Rx  variable_value=0  variable_type=uint8  numD=8  unitStr=""  descStr=""
      settings: AttributesFormatString=type:%<variable_type> Dimensions:%<numD>  SourceProductName=EcoCoder Blocks
  Write and Read Measurement1 : CoderSF_BSW_Libs/Calibration & Measurement/Write and Read Measurement  variable_name=LIN_Id4_RxRes  variable_value=0  variable_type=uint8  numD=1  unitStr=""  descStr=""
      settings: AttributesFormatString=type:%<variable_type> Dimensions:%<numD>  SourceProductName=EcoCoder Blocks
  wires:
  Write and Read Measurement/1 -> Subsystem/1(In1)
  Write and Read Measurement1/1 -> Subsystem/Trigger
  LIN Receive Data1/2 -> Write and Read Measurement/1
  LIN Receive Data1/1 -> Write and Read Measurement1/1

== system ECO_TestLibs/LINAMaster/RTX/Mst Rx send 0 ==
  Trigger : TriggerPort  VariantControl=(inherit)
  LIN Transmit Data2 : CoderSF_BSW_Libs/LIN/LIN Transmit Data  channel=LIN_A  Frame_Id=hex2dec('4')  Frame_Len=8  Frame_Dir=MasterReceive  Frame_CCS=Classic  Task_TimeIdx=Task_Inherit
      settings: SourceProductName=EcoCoder Blocks
  Read Calibration1 : CoderSF_BSW_Libs/Calibration & Measurement/Read Calibration  variable_name=send_data3  variable_value=[1,2,3,4,5,6,7,8]  variable_type=uint8  variable_min=[]  variable_max=[]  unitStr=""  descStr=""
      settings: AttributesFormatString=value:%<variable_value> type:%<variable_type> max:%<variable_max> Min:%<variable_min>  SourceProductName=EcoCoder Blocks
  wires:
  Read Calibration1/1 -> LIN Transmit Data2/1

== system ECO_TestLibs/LINAMaster/RTX/Mst send 0 ==
  Trigger : TriggerPort  VariantControl=(inherit)
  LIN Transmit Data1 : CoderSF_BSW_Libs/LIN/LIN Transmit Data  channel=LIN_A  Frame_Id=hex2dec('0')  Frame_Len=3  Frame_Dir=MasterSend  Frame_CCS=Enhanced  Task_TimeIdx=Task_Inherit
      settings: SourceProductName=EcoCoder Blocks
  Read Calibration1 : CoderSF_BSW_Libs/Calibration & Measurement/Read Calibration  variable_name=send_data0  variable_value=[1,2,3]  variable_type=uint8  variable_min=[]  variable_max=[]  unitStr=""  descStr=""
      settings: AttributesFormatString=value:%<variable_value> type:%<variable_type> max:%<variable_max> Min:%<variable_min>  SourceProductName=EcoCoder Blocks
  wires:
  Read Calibration1/1 -> LIN Transmit Data1/1

== system ECO_TestLibs/LINAMaster/RTX/Mst send 1 ==
  Trigger : TriggerPort  VariantControl=(inherit)
  LIN Transmit Data2 : CoderSF_BSW_Libs/LIN/LIN Transmit Data  channel=LIN_A  Frame_Id=hex2dec('1')  Frame_Len=3  Frame_Dir=MasterSend  Frame_CCS=Enhanced  Task_TimeIdx=Task_Inherit
      settings: SourceProductName=EcoCoder Blocks
  Read Calibration2 : CoderSF_BSW_Libs/Calibration & Measurement/Read Calibration  variable_name=send_data1  variable_value=[1,2,3]  variable_type=uint8  variable_min=[]  variable_max=[]  unitStr=""  descStr=""
      settings: AttributesFormatString=value:%<variable_value> type:%<variable_type> max:%<variable_max> Min:%<variable_min>  SourceProductName=EcoCoder Blocks
  wires:
  Read Calibration2/1 -> LIN Transmit Data2/1

== system ECO_TestLibs/LINAMaster/RTX/Mst send 2 ==
  Trigger : TriggerPort  VariantControl=(inherit)
  LIN Transmit Data2 : CoderSF_BSW_Libs/LIN/LIN Transmit Data  channel=LIN_A  Frame_Id=hex2dec('2')  Frame_Len=4  Frame_Dir=MasterSend  Frame_CCS=Classic  Task_TimeIdx=Task_Inherit
      settings: SourceProductName=EcoCoder Blocks
  Read Calibration1 : CoderSF_BSW_Libs/Calibration & Measurement/Read Calibration  variable_name=send_data2  variable_value=[1,2,3,4]  variable_type=uint8  variable_min=[]  variable_max=[]  unitStr=""  descStr=""
      settings: AttributesFormatString=value:%<variable_value> type:%<variable_type> max:%<variable_max> Min:%<variable_min>  SourceProductName=EcoCoder Blocks
  wires:
  Read Calibration1/1 -> LIN Transmit Data2/1

== system ECO_TestLibs/LINASlave/Rx/Subsystem ==
  In1 : Inport
  Enable : EnablePort
  1 : Constant  Value=0  OutDataTypeStr=Inherit: Inherit via back propagation
  2 : Constant  Value=0  OutDataTypeStr=Inherit: Inherit via back propagation
  3 : Constant  Value=hex2dec('210')  OutDataTypeStr=Inherit: Inherit via back propagation
  4 : Constant  Value=8  OutDataTypeStr=Inherit: Inherit via back propagation
  Demux : Demux  Outputs=3
  Transmit CAN Message : CoderSF_BSW_Libs/CAN/Transmit CAN Message  channel=CAN_C  tasktimeIndex=Task_Inherit
      settings: SourceProductName=EcoCoder Blocks
  Vector Concatenate : Concatenate  NumInputs=8
  Write Measurement : CoderSF_BSW_Libs/Calibration & Measurement/Write Measurement  variable_name=LIN_Rx0  variable_value=0  variable_type=uint8  numD=3  unitStr=""  descStr=""
      settings: AttributesFormatString=type:%<variable_type> Dimensions:%<numD>  SourceProductName=EcoCoder Blocks
  cntValue1 : Subsystem
  wires:
  In1/1 -> Demux/1, Write Measurement/1
  3/1 -> Transmit CAN Message/3
  4/1 -> Transmit CAN Message/4
  2/1 -> Transmit CAN Message/2
  1/1 -> Transmit CAN Message/1
  Vector Concatenate/1 -> Transmit CAN Message/5
  Demux/2 -> Vector Concatenate/2
  Demux/1 -> Vector Concatenate/1
  Demux/3 -> Vector Concatenate/3
  cntValue1/1(Out1) -> Vector Concatenate/4
  cntValue1/2(Out2) -> Vector Concatenate/5
  cntValue1/3(Out3) -> Vector Concatenate/6
  cntValue1/4(Out4) -> Vector Concatenate/7
  cntValue1/5(Out5) -> Vector Concatenate/8

== system ECO_TestLibs/LINASlave/Rx/Subsystem1 ==
  In1 : Inport
  Enable : EnablePort
  1 : Constant  Value=0  OutDataTypeStr=Inherit: Inherit via back propagation
  2 : Constant  Value=0  OutDataTypeStr=Inherit: Inherit via back propagation
  3 : Constant  Value=hex2dec('211')  OutDataTypeStr=Inherit: Inherit via back propagation
  4 : Constant  Value=8  OutDataTypeStr=Inherit: Inherit via back propagation
  Demux : Demux  Outputs=3
  Transmit CAN Message : CoderSF_BSW_Libs/CAN/Transmit CAN Message  channel=CAN_C  tasktimeIndex=Task_Inherit
      settings: SourceProductName=EcoCoder Blocks
  Vector Concatenate : Concatenate  NumInputs=8
  Write Measurement : CoderSF_BSW_Libs/Calibration & Measurement/Write Measurement  variable_name=LIN_Rx1  variable_value=0  variable_type=uint8  numD=3  unitStr=""  descStr=""
      settings: AttributesFormatString=type:%<variable_type> Dimensions:%<numD>  SourceProductName=EcoCoder Blocks
  cntValue1 : Subsystem
  wires:
  In1/1 -> Demux/1, Write Measurement/1
  3/1 -> Transmit CAN Message/3
  4/1 -> Transmit CAN Message/4
  2/1 -> Transmit CAN Message/2
  1/1 -> Transmit CAN Message/1
  Demux/2 -> Vector Concatenate/2
  Demux/1 -> Vector Concatenate/1
  Demux/3 -> Vector Concatenate/3
  Vector Concatenate/1 -> Transmit CAN Message/5
  cntValue1/1(Out1) -> Vector Concatenate/4
  cntValue1/2(Out2) -> Vector Concatenate/5
  cntValue1/3(Out3) -> Vector Concatenate/6
  cntValue1/4(Out4) -> Vector Concatenate/7
  cntValue1/5(Out5) -> Vector Concatenate/8
